simulink model "lab7_sfunc"  (R2018b)
settings: Solver=VariableStepAuto  StartTime=0.0  StopTime=10.0  RelTol=1e-3
settings Model: Creator=student  LastModifiedBy=student

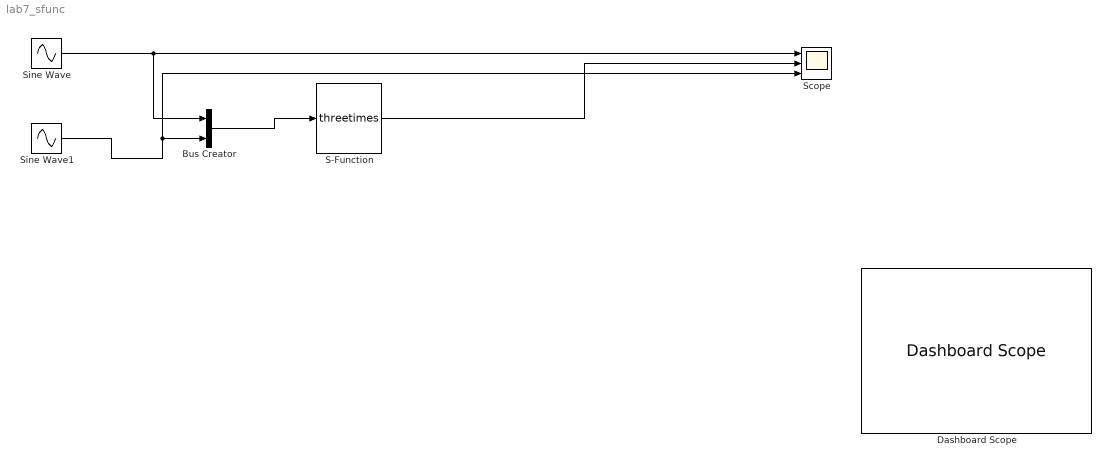
== system lab7_sfunc ==
  Bus Creator : BusCreator  Inputs=2
  Dashboard Scope : DashboardScope  WebBlockId=6
  S-Function : S-Function  FunctionName=threetimes  Parameters=3  SFunctionDeploymentMode=off  EnableBusSupport=off
      mask Display: image('C:\Users\student\Downloads\image.jpg');
  Scope : Scope  NumInputPorts=3
  Sine Wave : Sin  Amplitude=2  SampleTime=0
  Sine Wave1 : Sin  SampleTime=0
  wires:
  Sine Wave/1 -> Bus Creator/1, Scope/1
  Sine Wave1/1 -> Bus Creator/2, Scope/3
  Bus Creator/1 -> S-Function/1
  S-Function/1 -> Scope/2
